simulink model "Day6"  (R2021a)
settings: Solver=VariableStepAuto  StartTime=0.0  StopTime=10.0  RelTol=1e-3
values from neighbouring files (symbols this model uses):
  l1 = input('enter value for link1: ')    [Day10.m]    (also in Day8.m = input('Enter link 1: '); LabFile9.m = 10)
  l2 = input('enter value for link2: ')    [Day10.m]    (also in Day8.m = input('Enter link 2: '); LabFile9.m = 20)
settings Model: Creator=Kanha  LastModifiedBy=Kanha

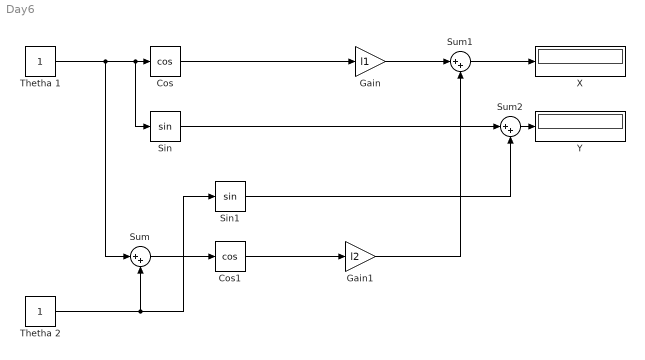
== system Day6 ==
  Cos : Trigonometry  Operator=cos
  Cos1 : Trigonometry  Operator=cos
  Gain : Gain  Gain=l1
  Gain1 : Gain  Gain=l2
  Sin : Trigonometry
  Sin1 : Trigonometry
  Sum : Sum  Inputs=|++
  Sum1 : Sum  Inputs=|++
  Sum2 : Sum  Inputs=|++
  Thetha 1 : Constant
  Thetha 2 : Constant
  X : Display
  Y : Display
  wires:
  Thetha 1/1 -> Sum/1, Sin/1, Cos/1
  Cos/1 -> Gain/1
  Thetha 2/1 -> Sin1/1, Sum/2
  Sum/1 -> Cos1/1
  Cos1/1 -> Gain1/1
  Gain/1 -> Sum1/1
  Gain1/1 -> Sum1/2
  Sum1/1 -> X/1
  Sin/1 -> Sum2/1
  Sin1/1 -> Sum2/2
  Sum2/1 -> Y/1
